simulink model "SynchGenerator_SimplifiedModel"  (R2016b)
settings: Solver=FixedStepAuto  StartTime=0.0  StopTime=0.3  FixedStep=0.0001  RelTol=1e-3
values from neighbouring files (symbols this model uses):
  Lmd_pu = Lmd/Lsbase    (= 1.65989189445)    [param_SynchGenerator_Kundur_3_1.m]    (also in param_SynchGenerator_Kundur_3_1_mathworks.m)
  Rf_pu = Rf/Zfbase    (= 0.000599873078326)    [param_SynchGenerator_Kundur_3_1.m]    (also in param_SynchGenerator_Kundur_3_1_mathworks.m)
undefined symbols (not defined in the file or in its folder): pe
libraries: pe_lib x7, nesl_utility x7, fl_lib x6
settings Model: Creator=mmi-vsa  LastModifiedBy=mmi-vsa

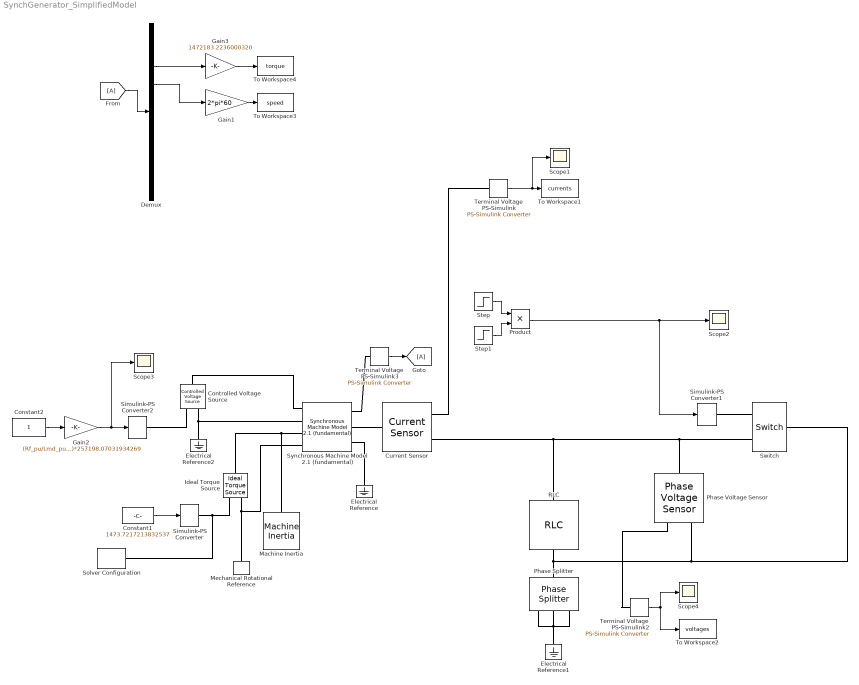
== system SynchGenerator_SimplifiedModel ==
  Constant1 : Constant  Value=1473.7217213832537
  Constant2 : Constant
  Controlled Voltage Source : fl_lib/Electrical/Electrical Sources/Controlled Voltage Source
  Current Sensor : pe_lib/Sensors/Current Sensor
  Demux : Demux  Outputs=10
  Electrical Reference : fl_lib/Electrical/Electrical Elements/Electrical Reference
  Electrical Reference1 : fl_lib/Electrical/Electrical Elements/Electrical Reference
  Electrical Reference2 : fl_lib/Electrical/Electrical Elements/Electrical Reference
  Gain1 : Gain  Gain=2*pi*60
  Gain2 : Gain  Gain=(Rf_pu/Lmd_pu)*257198.07031934269
  Gain3 : Gain  Gain=1472183.2236000320
  Ideal Torque Source : fl_lib/Mechanical/Mechanical Sources/Ideal Torque Source
  Machine Inertia : pe_lib/Machines/Machine Inertia  SRated=555e6 V*A  FRated=60 Hz  nPolePairs=1  inertia_option=2  J=27548 kg*m^2  H=3.7 s*W/V/A  damper_option=2  D=39.0509 N*m/(rad/s)  pu_D=0  initialization_option=2  fMechanical0=60 Hz  fElectrical0=60 Hz
  Mechanical Rotational Reference : fl_lib/Mechanical/Rotational Elements/Mechanical Rotational Reference
  Phase Splitter : pe_lib/Connections/Phase Splitter
  Phase Voltage Sensor : pe_lib/Sensors/Phase Voltage Sensor
  Product : Product
  RLC : pe_lib/Passive Devices/RLC  component_structure=1  R=1.92 - 0.001 Ohm  L=0.001 H  IL0=[ 0 0 0 ] A  C=1e-6 F  VC0=[ 0 0 0 ] V  R_parasitic=1e-6 Ohm  G_parasitic=1e-6 1/Ohm
  Scope{1..4} (4 alike) : Scope
  Simulink-PS Converter : nesl_utility/Simulink-PS Converter  PhysicalDomain=network_engine_domain  SubClassName=ps_input  LeftPortType=input  RightPortType=output  PseudoPeriodic=off  Frequencies=[]  NoiseDistribution=none  NoiseParameters=[]  Unit=1  AffineConversion=off  InputFiltering=off  SimscapeFilterOrder=1  InputFilterTimeConstant=0.001  UdotUserProvided=1
  Simulink-PS Converter1 : nesl_utility/Simulink-PS Converter  PhysicalDomain=network_engine_domain  SubClassName=ps_input  LeftPortType=input  RightPortType=output  PseudoPeriodic=off  Frequencies=[]  NoiseDistribution=none  NoiseParameters=[]  Unit=1  AffineConversion=off  InputFiltering=off  SimscapeFilterOrder=1  InputFilterTimeConstant=0.001  UdotUserProvided=1
  Simulink-PS Converter2 : nesl_utility/Simulink-PS Converter  PhysicalDomain=network_engine_domain  SubClassName=ps_input  LeftPortType=input  RightPortType=output  PseudoPeriodic=off  Frequencies=[]  NoiseDistribution=none  NoiseParameters=[]  Unit=1  AffineConversion=off  InputFiltering=off  SimscapeFilterOrder=1  InputFilterTimeConstant=0.001  UdotUserProvided=1
  Solver Configuration : nesl_utility/Solver Configuration  PhysicalDomain=network_engine_domain  SubClassName=solver  LeftPortType=input  RightPortType=generic  Accelerate=off  Tones=[]  Harmonics=[]  SimulateNoise=off  Profile=off  UseLocalSampling=off  EnableSwitchedLinearOptims=on  FrequencyDomain=off  UseCCode=off  RelTol=0.001  AbsTol=1e-06  MinStep=1e-09  ToWorkspace=off  RevertToSquareIcSolve=off  NumHomotopyIterations=100  PhasorMode=off  PhasorModeNumHarmonics=1  OverrideAbsTol=off  DoDC=off  ResidualTolerance=1e-09  UseLocalSolver=on  LocalSolverChoice=NE_TRAPEZOIDAL_ADVANCER  LocalSolverSampleTime=1e-4  DoFixedCost=on  MaxNonlinIter=3  MaxModeIter=2  LinearAlgebra=Sparse  DelaysMemoryBudget=1024  AutomaticFiltering=off  FilteringTimeConstant=0.001
  Step : Step  Time=0.1  SampleTime=0
  Step1 : Step  Time=0.2  Before=1  After=0  SampleTime=0
  Switch : pe_lib/Switches & Breakers/Switch  R_closed=0.001 Ohm  G_open=1e-12 1/Ohm  threshold=0.5 V  i_vT_specify=off  i_vT_priority=None  i_vT=0 A  I_specify=off  I_priority=None  I=[ 0 0 0 ] A  V_specify=off  V_priority=None  V=[ 0 0 0 ] V  i_a_specify=off  i_a_priority=None  i_a=0 A  v_a_specify=off  v_a_priority=None  v_a=0 V  i_b_specify=off  i_b_priority=None  i_b=0 A  v_b_specify=off  v_b_priority=None  v_b=0 V  i_c_specify=off  i_c_priority=None  i_c=0 A  v_c_specify=off  v_c_priority=None  v_c=0 V
  Synchronous Machine Model 2.1 (fundamental) : pe_lib/Machines/Synchronous Machine (Simplified)/Synchronous Machine Model 2.1 (fundamental)  SRated=555e6 V*A  VRated=24e3 V  FRated=60 Hz  nPolePairs=1  fieldCircuitParameterization_option=2  baseEfd=92.95 V  baseIfd=1300 A  Ladu=Lmd_pu  Laqu=Lmq_pu  Ll=Ll_pu  Ra=Rs_pu  Lfd=Llfd_pu  Rfd=Rf_pu  L1d=Llkd_pu  R1d=Rkd_pu  L1q=Llkq1_pu  R1q=Rkq2_pu  initialization_option=2  angular_position0=0 deg  eddd0=0  eqd0=0  eqdd0=0  Vmag0=24000 V  Vang0=-pi rad  Pt0=300e6 W  Qt0=0 V*A  shift_3ph=[nan, nan, nan] rad  connection_option=int32(pe.Connection.wye)  num_q_dampers=1  Xl=nan  Xd=nan  Xq=nan  Xdd=nan  Xddd=nan  Xqdd=nan  Td0d=nan s  Td0dd=nan s  Tq0dd=nan s  base_v=nan V  base_i=nan A  base_torque=nan N*m  base_wMechanical=nan rad/s  base_rc_efd=nan V  base_rc_ifd=nan A  base_fd_Efd=nan V  base_fd_Ifd=nan A
  Terminal Voltage PS-Simulink : nesl_utility/PS-Simulink Converter  PhysicalDomain=network_engine_domain  SubClassName=ps_output  LeftPortType=input  RightPortType=output  PseudoPeriodic=off  Frequencies=[]  Unit=1  AffineConversion=off
  Terminal Voltage PS-Simulink2 : nesl_utility/PS-Simulink Converter  PhysicalDomain=network_engine_domain  SubClassName=ps_output  LeftPortType=input  RightPortType=output  PseudoPeriodic=off  Frequencies=[]  Unit=1  AffineConversion=off
  Terminal Voltage PS-Simulink3 : nesl_utility/PS-Simulink Converter  PhysicalDomain=network_engine_domain  SubClassName=ps_output  LeftPortType=input  RightPortType=output  PseudoPeriodic=off  Frequencies=[]  Unit=1  AffineConversion=off
  To Workspace1 : ToWorkspace  VariableName=currents  SampleTime=-1
  To Workspace2 : ToWorkspace  VariableName=voltages  SampleTime=-1
  To Workspace3 : ToWorkspace  VariableName=speed  SampleTime=-1
  To Workspace4 : ToWorkspace  VariableName=torque  SampleTime=-1
  wires:
  Terminal Voltage PS-Simulink/1 -> Scope1/1, To Workspace1/1
  Constant1/1 -> Simulink-PS Converter/1
  Terminal Voltage PS-Simulink2/1 -> Scope4/1, To Workspace2/1
  Terminal Voltage PS-Simulink3/1 -> [A]
  [A] -> Demux/1
  Gain2/1 -> Scope3/1, Simulink-PS Converter2/1
  Gain1/1 -> To Workspace3/1
  Demux/4 -> Gain1/1
  Gain3/1 -> To Workspace4/1
  Demux/3 -> Gain3/1
  Constant2/1 -> Gain2/1
  Step/1 -> Product/1
  Step1/1 -> Product/2
  Product/1 -> Simulink-PS Converter1/1, Scope2/1
  connections:
  Mechanical Rotational Reference/LConn1 -- Synchronous Machine Model 2.1 (fundamental)/LConn4 -- Ideal Torque Source/RConn2
  Ideal Torque Source/LConn1 -- Synchronous Machine Model 2.1 (fundamental)/LConn3 -- Machine Inertia/LConn1
  Simulink-PS Converter/RConn1 -- Solver Configuration/RConn1 -- Ideal Torque Source/RConn1
  Electrical Reference/LConn1 -- Synchronous Machine Model 2.1 (fundamental)/RConn3
  Simulink-PS Converter2/RConn1 -- Controlled Voltage Source/RConn1
  Synchronous Machine Model 2.1 (fundamental)/RConn2 -- Current Sensor/LConn1
  Terminal Voltage PS-Simulink/LConn1 -- Current Sensor/RConn1
  Phase Voltage Sensor/LConn1 -- Current Sensor/RConn2 -- RLC/LConn1 -- Switch/LConn2
  Simulink-PS Converter1/RConn1 -- Switch/LConn1
  Electrical Reference1/LConn1 -- Phase Splitter/RConn3 -- Phase Splitter/RConn1 -- Phase Splitter/RConn2
  Terminal Voltage PS-Simulink2/LConn1 -- Phase Voltage Sensor/RConn1
  Synchronous Machine Model 2.1 (fundamental)/RConn1 -- Terminal Voltage PS-Simulink3/LConn1
  Controlled Voltage Source/LConn1 -- Synchronous Machine Model 2.1 (fundamental)/LConn1
  Controlled Voltage Source/RConn2 -- Electrical Reference2/LConn1 -- Synchronous Machine Model 2.1 (fundamental)/LConn2
  Phase Splitter/LConn1 -- Switch/RConn1 -- Phase Voltage Sensor/RConn2 -- RLC/RConn1
